simulink model "TP3"  (R2024b)
settings: Solver=ode23t  StartTime=0.0  StopTime=4  RelTol=1e-3
InitFcn:
  | parametretp3
StartFcn:
  | parametretp3
values from neighbouring files (symbols this model uses):
  Cr = 0    [parametretp3.m]
  J = 3.2284e-6    (= 3.2284e-06)    [parameters.m]    (also in parametretp3.m = 0.2)
  L = 2.75e-6    (= 2.75e-06)    [parameters.m]    (also in parametretp3.m = 0.012161)
  p = 3    [parametretp3.m]
  psi = pi/4    (= 0.785398163397)    [parametretp3.m]
  R = 4    [parameters.m]    (also in parametretp3.m = 0.895)
  tetaf = K/p    (= 0.3)    [parametretp3.m]
  U0 = 220    [parametretp3.m]
settings Model: Creator=E306-PC5  LastModifiedBy=E306-PC5

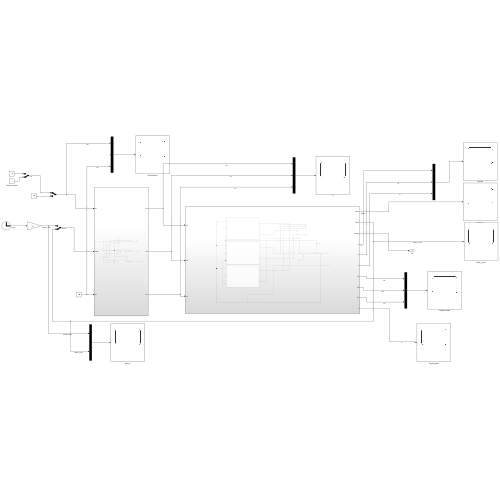
[thumbnail: Simulink's stored preview of the top-level diagram]
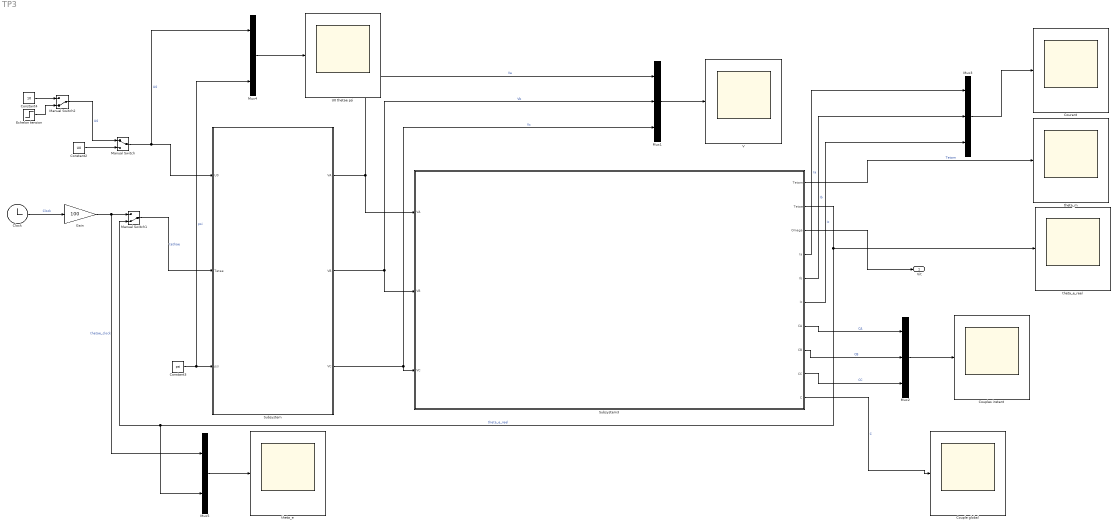
== system TP3 ==
  Clock : Clock
  Constant2 : Constant  Value=U0
  Constant3 : Constant  Value=psi
  Constant4 : Constant  Value=10
  Couple global : Scope
  Couples instant : Scope
  Courant : Scope
  Echelon tension : Step  After=10  SampleTime=0
  Gain : Gain  Gain=100
  Manual Switch : ManualSwitch
  Manual Switch1 : ManualSwitch  CurrentSetting=0
  Manual Switch2 : ManualSwitch  CurrentSetting=0
  Mux{1..4} (4 alike) : Mux  Inputs=3
  Mux5 : Mux  Inputs=2
  Subsystem : Subsystem
  Subsystem3 : Subsystem
  U0 thetae psi : Scope
  V : Scope
  theta_e : Scope
  theta_e_reel : Scope
  theta_m : Scope
  Vit : Outport
  wires:
  Clock/1 -> Gain/1  "Clock"
  Mux1/1 -> V/1
  Subsystem3/2(Tetae) -> Mux5/2, Manual Switch1/2, theta_e_reel/1  "theta_e_reel"
  Subsystem3/1(Tetam) -> theta_m/1  "Tetam"
  Mux3/1 -> Courant/1
  Subsystem3/4(Ia) -> Mux3/1  "Ia"
  Subsystem3/5(Ib) -> Mux3/2  "Ib"
  Subsystem3/6(Ic) -> Mux3/3  "Ic"
  Subsystem/2(VB) -> Mux1/2, Subsystem3/2(VB)  "Vb"
  Subsystem/1(VA) -> Mux1/1, Subsystem3/1(VA)  "Va"
  Subsystem/3(VC) -> Mux1/3, Subsystem3/3(VC)  "Vc"
  Manual Switch/1 -> Mux4/1, Subsystem/1(U0)  "U0"
  Constant3/1 -> Mux4/3, Subsystem/3(psi)  "psi"
  Mux4/1 -> U0 thetae psi/1
  Gain/1 -> Mux5/1, Manual Switch1/1  "thetae_clock"
  Manual Switch1/1 -> Subsystem/2(Tetae)  "tethae"
  Mux5/1 -> theta_e/1
  Subsystem3/3(Omega) -> Vit/1
  Constant2/1 -> Manual Switch/2
  Manual Switch2/1 -> Manual Switch/1  "U0"
  Constant4/1 -> Manual Switch2/1
  Echelon tension/1 -> Manual Switch2/2
  Mux2/1 -> Couples instant/1
  Subsystem3/7(CA) -> Mux2/1  "CA"
  Subsystem3/8(CB) -> Mux2/2  "CB"
  Subsystem3/9(CC) -> Mux2/3  "CC"
  Subsystem3/10(C) -> Couple global/1  "C"

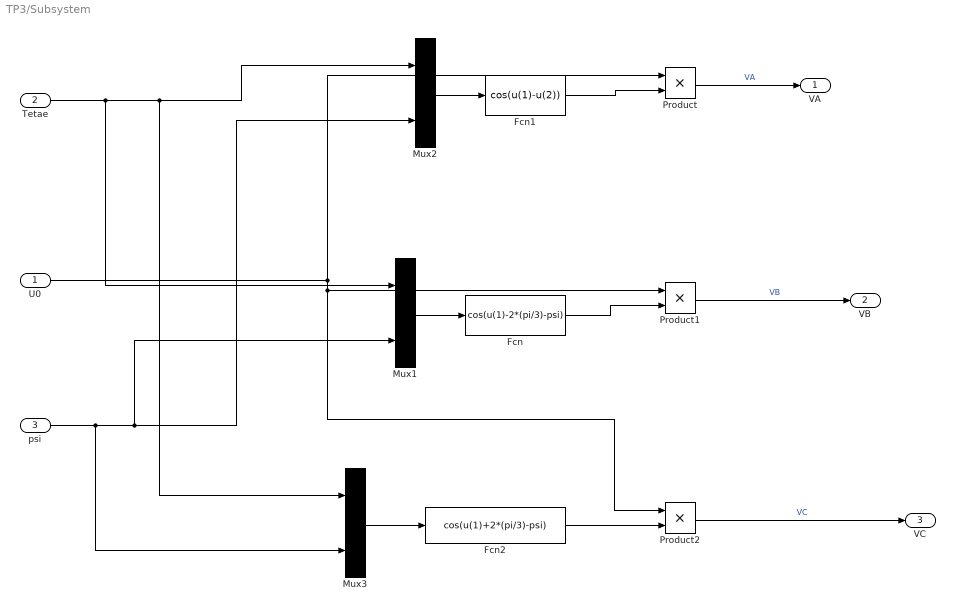
== system TP3/Subsystem ==
  U0 : Inport
  Tetae : Inport  Port=2
  psi : Inport  Port=3
  Fcn : Fcn  Expr=cos(u(1)-2*(pi/3)-psi)
  Fcn1 : Fcn  Expr=cos(u(1)-u(2))
  Fcn2 : Fcn  Expr=cos(u(1)+2*(pi/3)-psi)
  Mux1 : Mux  Inputs=2
  Mux2 : Mux  Inputs=2
  Mux3 : Mux  Inputs=2
  Product : Product
  Product1 : Product
  Product2 : Product
  VA : Outport
  VB : Outport  Port=2
  VC : Outport  Port=3
  wires:
  Fcn1/1 -> Product/2
  Product2/1 -> VC/1  "VC"
  Tetae/1 -> Mux1/1, Mux3/1, Mux2/1
  U0/1 -> Product2/1, Product1/1, Product/1
  Product1/1 -> VB/1  "VB"
  Fcn/1 -> Product1/2
  Fcn2/1 -> Product2/2
  Product/1 -> VA/1  "VA"
  psi/1 -> Mux3/2, Mux2/2, Mux1/2
  Mux2/1 -> Fcn1/1
  Mux1/1 -> Fcn/1
  Mux3/1 -> Fcn2/1

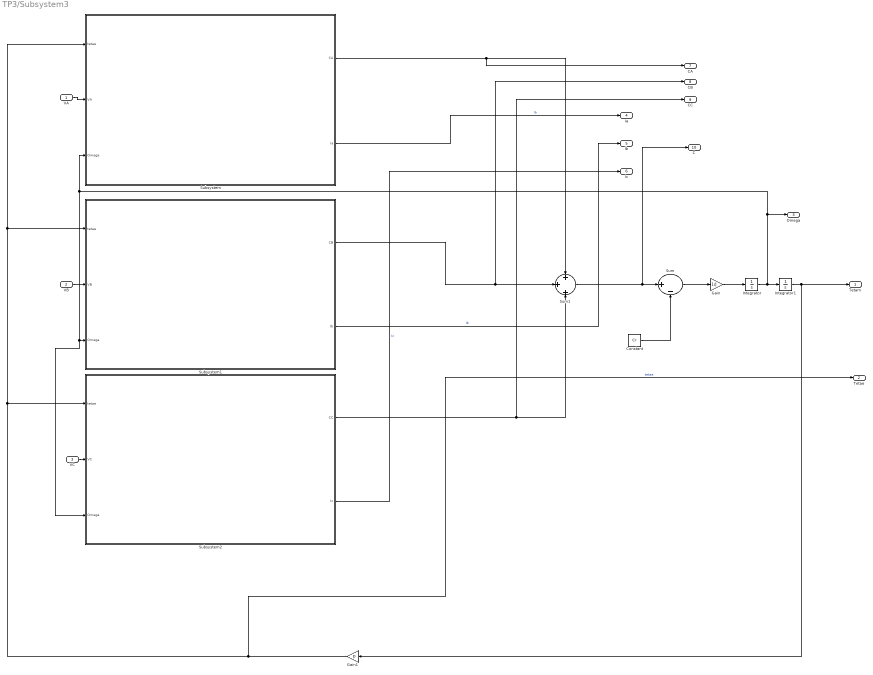
== system TP3/Subsystem3 ==
  VA : Inport
  VB : Inport  Port=2
  VC : Inport  Port=3
  Constant : Constant  Value=Cr
  Gain : Gain  Gain=1/J
  Gain1 : Gain  Gain=p
  Integrator : Integrator
  Integrator1 : Integrator
  Subsystem : Subsystem
  Subsystem1 : Subsystem
  Subsystem2 : Subsystem
  Sum : Sum  Inputs=|+-
  Sum1 : Sum  Inputs=+|+|+
  Tetam : Outport
  Tetae : Outport  Port=2
  Omega : Outport  Port=3
  Ia : Outport  Port=4
  Ib : Outport  Port=5
  Ic : Outport  Port=6
  CA : Outport  Port=7
  CB : Outport  Port=8
  CC : Outport  Port=9
  C : Outport  Port=10
  wires:
  Integrator/1 -> Omega/1, Subsystem2/3(Omega), Subsystem1/3(Omega), Subsystem/3(Omega), Integrator1/1
  Gain1/1 -> Tetae/1, Subsystem/1(tetae), Subsystem1/1(tetae), Subsystem2/1(tetae)  "tetae"
  Gain/1 -> Integrator/1
  Subsystem/1(CA) -> CA/1, Sum1/1
  Sum/1 -> Gain/1
  Sum1/1 -> C/1, Sum/1
  Subsystem1/1(CB) -> CB/1, Sum1/2
  Constant/1 -> Sum/2
  Integrator1/1 -> Tetam/1, Gain1/1
  VA/1 -> Subsystem/2(VA)
  VB/1 -> Subsystem1/2(VB)
  VC/1 -> Subsystem2/2(VC)
  Subsystem2/1(CC) -> CC/1, Sum1/3
  Subsystem/2(Ia) -> Ia/1  "Ia"
  Subsystem1/2(Ib) -> Ib/1  "Ib"
  Subsystem2/2(Ic) -> Ic/1  "Ic"

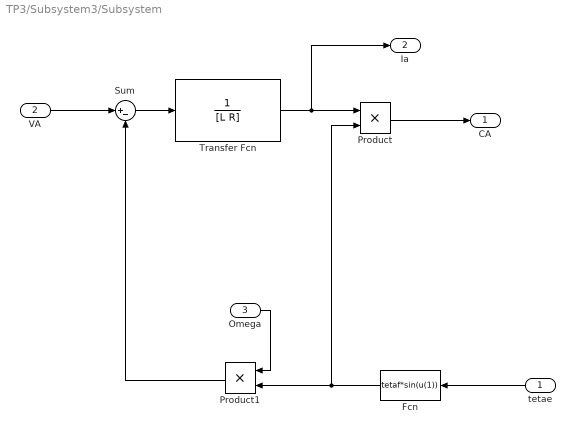
== system TP3/Subsystem3/Subsystem ==
  tetae : Inport
  VA : Inport  Port=2
  Omega : Inport  Port=3
  Fcn : Fcn  Expr=tetaf*sin(u(1))
  Product : Product
  Product1 : Product
  Sum : Sum  Inputs=|+-
  Transfer Fcn : TransferFcn  Denominator=[L R]
  CA : Outport
  Ia : Outport  Port=2
  wires:
  Transfer Fcn/1 -> Ia/1, Product/1
  Product/1 -> CA/1
  Product1/1 -> Sum/2
  Fcn/1 -> Product/2, Product1/2
  VA/1 -> Sum/1
  tetae/1 -> Fcn/1
  Sum/1 -> Transfer Fcn/1
  Omega/1 -> Product1/1

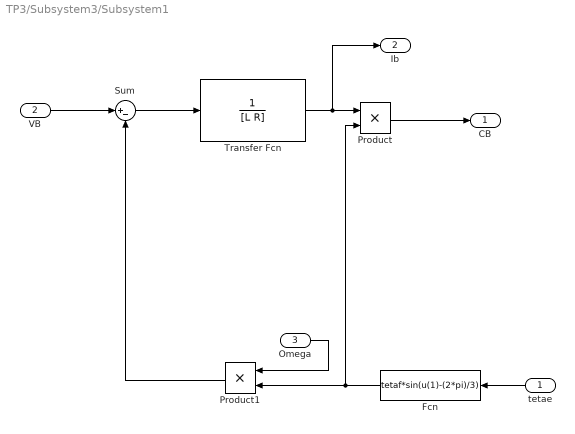
== system TP3/Subsystem3/Subsystem1 ==
  tetae : Inport
  VB : Inport  Port=2
  Omega : Inport  Port=3
  Fcn : Fcn  Expr=tetaf*sin(u(1)-(2*pi)/3)
  Product : Product
  Product1 : Product
  Sum : Sum  Inputs=|+-
  Transfer Fcn : TransferFcn  Denominator=[L R]
  CB : Outport
  Ib : Outport  Port=2
  wires:
  Transfer Fcn/1 -> Ib/1, Product/1
  Product/1 -> CB/1
  Product1/1 -> Sum/2
  Fcn/1 -> Product1/2, Product/2
  VB/1 -> Sum/1
  tetae/1 -> Fcn/1
  Sum/1 -> Transfer Fcn/1
  Omega/1 -> Product1/1

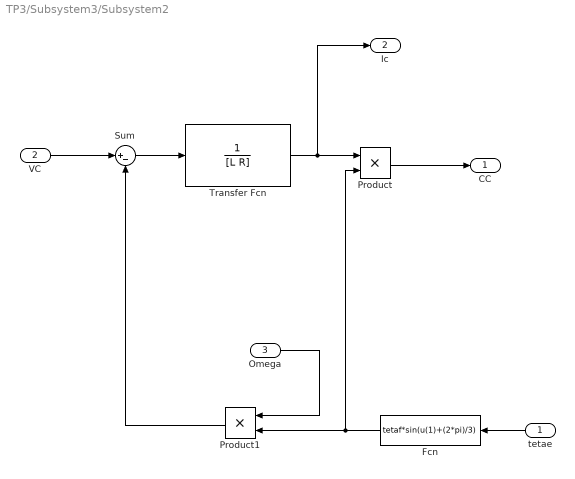
== system TP3/Subsystem3/Subsystem2 ==
  tetae : Inport
  VC : Inport  Port=2
  Omega : Inport  Port=3
  Fcn : Fcn  Expr=tetaf*sin(u(1)+(2*pi)/3)
  Product : Product
  Product1 : Product
  Sum : Sum  Inputs=|+-
  Transfer Fcn : TransferFcn  Denominator=[L R]
  CC : Outport
  Ic : Outport  Port=2
  wires:
  Transfer Fcn/1 -> Ic/1, Product/1
  Product/1 -> CC/1
  Product1/1 -> Sum/2
  Fcn/1 -> Product1/2, Product/2
  VC/1 -> Sum/1
  tetae/1 -> Fcn/1
  Sum/1 -> Transfer Fcn/1
  Omega/1 -> Product1/1
